simulink model "viswa9"  (Simulink 7.3)
settings: Solver=ode45  StartTime=0.0  StopTime=0.5  RelTol=1e-3
undefined symbols (not defined in the file): D11, Delta, Hydride, magnitude, Metal, Nickel
libraries: powerlib x34, powerlib_extras x3, electricdrivelib x2, powerlib_models x2, simulink x1
settings Model: Creator=KREST  LastModifiedBy=s padmaja

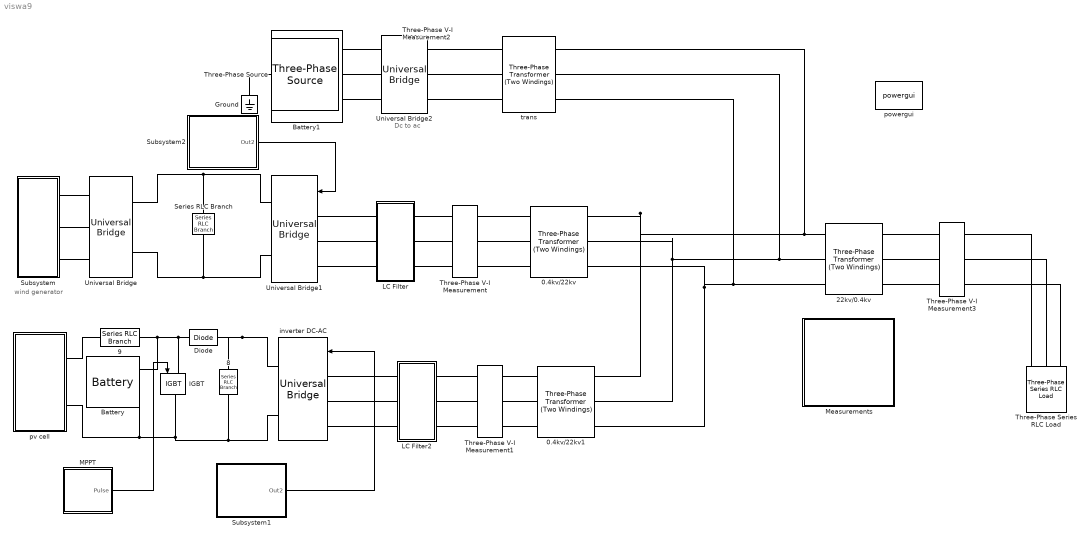
== system viswa9 ==
  note: Dc to ac
  note: wind generator
  0.4kv/22kv : powerlib/Elements/Three-Phase Transformer (Two Windings)  DialogController=POWERSYS.PowerSysDialog  SystemSampleTime=-1  Winding1Connection=Yg  UNITS=pu  NominalPower=[ 500e3 , 50 ]  Winding1=[ 0.4e3 , 0.002 , 0.08 ]  Winding2Connection=Delta (D11)  Winding2=[ 22e3 , 0.002 , 0.08 ]  SetSaturation=off  Rm=500  Lm=500  Saturation=[ 0,0 ; 0.0024,1.2 ; 1.0,1.52 ]  Hysteresis=off  DataFile='hysteresis'  SetInitialFlux=off  InitialFluxes=[ 0.8 , -0.8 , 0.7 ]  Measurements=None  MoreParameters=off  BreakLoop=off  DataType=off  TransfoNumber=1
  0.4kv/22kv1 : powerlib/Elements/Three-Phase Transformer (Two Windings)  DialogController=POWERSYS.PowerSysDialog  SystemSampleTime=-1  Winding1Connection=Yg  UNITS=pu  NominalPower=[ 500e3 , 50 ]  Winding1=[ 0.4e3 , 0.002 , 0.08 ]  Winding2Connection=Delta (D11)  Winding2=[ 22e3 , 0.002 , 0.08 ]  SetSaturation=off  Rm=500  Lm=500  Saturation=[ 0,0 ; 0.0024,1.2 ; 1.0,1.52 ]  Hysteresis=off  DataFile='hysteresis'  SetInitialFlux=off  InitialFluxes=[ 0.8 , -0.8 , 0.7 ]  Measurements=None  MoreParameters=off  BreakLoop=off  DataType=off  TransfoNumber=1
  22kv/0.4kv : powerlib/Elements/Three-Phase Transformer (Two Windings)  DialogController=POWERSYS.PowerSysDialog  SystemSampleTime=-1  Winding1Connection=Delta (D11)  UNITS=pu  NominalPower=[ 500e3 , 50 ]  Winding1=[ 0.4e3 , 0.002 , 0.08 ]  Winding2Connection=Yg  Winding2=[ 22e3 , 0.002 , 0.08 ]  SetSaturation=off  Rm=500  Lm=500  Saturation=[ 0,0 ; 0.0024,1.2 ; 1.0,1.52 ]  Hysteresis=off  DataFile='hysteresis'  SetInitialFlux=off  InitialFluxes=[ 0.8 , -0.8 , 0.7 ]  Measurements=None  MoreParameters=off  BreakLoop=off  DataType=off  TransfoNumber=1
  8 : powerlib/Elements/Series RLC Branch  DialogController=POWERSYS.PowerSysDialog  PhysicalDomain=powersysdomain  SubClassName=unknown  LeftPortType=p1  RightPortType=p1  LConnTagsString=__new0  RConnTagsString=__new0  BranchType=C  Resistance=1  Inductance=1e-3  SetiL0=off  InitialCurrent=0  Capacitance=1e-6  Setx0=off  InitialVoltage=0  Measurements=None
  9 : powerlib/Elements/Series RLC Branch  DialogController=POWERSYS.PowerSysDialog  PhysicalDomain=powersysdomain  SubClassName=unknown  LeftPortType=p1  RightPortType=p1  LConnTagsString=__new0  RConnTagsString=__new0  BranchType=L  Resistance=1  Inductance=1e-3  SetiL0=off  InitialCurrent=0  Capacitance=1e-6  Setx0=off  InitialVoltage=0  Measurements=None
  Battery : electricdrivelib/Extra Sources/Battery  SystemSampleTime=-1  BatType=Nickel-Metal-Hydride  ShowDetailedParameters=off  NomV=1.2  NomQ=1.5  SOC=100  PresetModel=off  MaxQ=1.575  FullV=0.016963  Dis_rate=0.0045  R=0.008  Normal_OP=0.021635  expZone="[0.01562      0.0045]"  Dis_Char=off  current=[1.5 3]  Units=Ampere-hour  Batt_Tr=30
  Battery1 : electricdrivelib/Extra Sources/Battery  SystemSampleTime=-1  BatType=Nickel-Metal-Hydride  ShowDetailedParameters=off  NomV=1.2  NomQ=1.5  SOC=100  PresetModel=off  MaxQ=1.575  FullV=0.016963  Dis_rate=0.0045  R=0.008  Normal_OP=0.021635  expZone="[0.01562      0.0045]"  Dis_Char=off  current=[1.5 3]  Units=Ampere-hour  Batt_Tr=30
  Diode : powerlib/Power Electronics/Diode  DialogController=POWERSYS.PowerSysDialog  SystemSampleTime=-1  Ron=0.001  Lon=0  Vf=0.8  IC=0  UseSnubber=off  Rs=500  Cs=250e-9  Measurements=off
  Ground : powerlib/Elements/Ground  DialogController=POWERSYS.PowerSysDialog  PhysicalDomain=powersysdomain  SubClassName=unknown  LeftPortType=p1  RightPortType=p1  LConnTagsString=a
  IGBT : powerlib/Power Electronics/IGBT  DialogController=POWERSYS.PowerSysDialog  SystemSampleTime=-1  Ron=0.001  Lon=0  Vf=1  Tf=1e-6  Tt=2e-6  IC=0  Rs=1e5  Cs=inf  Measurements=off
  LC Filter : Subsystem
  LC Filter2 : Subsystem
  MPPT : Subsystem
  Measurements : Subsystem
  Series RLC Branch : powerlib/Elements/Series RLC Branch  DialogController=POWERSYS.PowerSysDialog  PhysicalDomain=powersysdomain  SubClassName=unknown  LeftPortType=p1  RightPortType=p1  LConnTagsString=__new0  RConnTagsString=__new0  BranchType=C  Resistance=1  Inductance=1e-3  SetiL0=off  InitialCurrent=0  Capacitance=600e-6  Setx0=off  InitialVoltage=0  Measurements=None
  Subsystem : Subsystem
  Subsystem1 : Subsystem
  Subsystem2 : Subsystem
  Three-Phase Series RLC Load : powerlib/Elements/Three-Phase Series RLC Load  DialogController=POWERSYS.PowerSysDialog  PhysicalDomain=powersysdomain  SubClassName=unknown  LeftPortType=p1  RightPortType=p1  LConnTagsString=A|B|C  Configuration=Y (grounded)  NominalVoltage=380  NominalFrequency=50  ActivePower=500e3  InductivePower=0  CapacitivePower=0  Measurements=None
  Three-Phase V-I Measurement : powerlib/Measurements/Three-Phase V-I Measurement  DialogController=POWERSYS.PowerSysDialog  SystemSampleTime=-1  VoltageMeasurement=phase-to-ground  SetLabelV=on  LabelV=Vhabc  Vpu=off  CurrentMeasurement=yes  SetLabelI=on  LabelI=Ihabc  Ipu=off  Pbase=100e6  Vbase=500e3  OutputType=Complex  PhasorSimulation=off  PSBequivalent=0
  Three-Phase V-I Measurement1 : powerlib/Measurements/Three-Phase V-I Measurement  DialogController=POWERSYS.PowerSysDialog  SystemSampleTime=-1  VoltageMeasurement=phase-to-ground  SetLabelV=on  LabelV=Vpvabc  Vpu=off  CurrentMeasurement=yes  SetLabelI=on  LabelI=Ipvabc  Ipu=off  Pbase=100e6  Vbase=500e3  OutputType=Complex  PhasorSimulation=off  PSBequivalent=0
  Three-Phase V-I Measurement2 : powerlib/Measurements/Three-Phase V-I Measurement  DialogController=POWERSYS.PowerSysDialog  SystemSampleTime=-1  VoltageMeasurement=phase-to-ground  SetLabelV=on  LabelV=VEabc  Vpu=off  CurrentMeasurement=yes  SetLabelI=on  LabelI=IEabc  Ipu=off  Pbase=100e6  Vbase=500e3  OutputType=Complex  PhasorSimulation=off  PSBequivalent=0
  Three-Phase V-I Measurement3 : powerlib/Measurements/Three-Phase V-I Measurement  DialogController=POWERSYS.PowerSysDialog  SystemSampleTime=-1  VoltageMeasurement=phase-to-ground  SetLabelV=on  LabelV=Vlabc  Vpu=off  CurrentMeasurement=yes  SetLabelI=on  LabelI=Ilabc  Ipu=off  Pbase=100e6  Vbase=500e3  OutputType=Complex  PhasorSimulation=off  PSBequivalent=0
  Three-Phase Source : powerlib/Electrical Sources/Three-Phase Source  DialogController=POWERSYS.PowerSysDialog  SystemSampleTime=-1  Voltage=132e3  PhaseAngle=0  Frequency=50  InternalConnection=Yn  SpecifyImpedance=on  Resistance=0.8929  Inductance=16.58e-3  ShortCircuitLevel=100e6  BaseVoltage=22e3  XRratio=7
  Universal Bridge : powerlib/Power Electronics/Universal Bridge  DialogController=POWERSYS.PowerSysDialog  SystemSampleTime=-1  Arms=3  SnubberResistance=1e5  SnubberCapacitance=inf  Device=Diodes  Ron=1e-3  Lon=0  ForwardVoltages="[  0  0  ]"  ForwardVoltage=0  GTOparameters=[ 10e-6 , 20e-6 ]  IGBTparameters=[ 1e-6 , 2e-6 ]  Measurements=None  Measurements_2=None  converterType=Rectifier
  Universal Bridge1 : powerlib/Power Electronics/Universal Bridge  DialogController=POWERSYS.PowerSysDialog  SystemSampleTime=-1  Arms=3  SnubberResistance=1e5  SnubberCapacitance=inf  Device=IGBT / Diodes  Ron=1e-3  Lon=0  ForwardVoltages="[  0  0  ]"  ForwardVoltage=0  GTOparameters=[ 10e-6 , 20e-6 ]  IGBTparameters=[ 1e-6 , 2e-6 ]  Measurements=None  Measurements_2=None  converterType=Rectifier
  Universal Bridge2 : powerlib/Power Electronics/Universal Bridge  DialogController=POWERSYS.PowerSysDialog  SystemSampleTime=-1  Arms=3  SnubberResistance=1e5  SnubberCapacitance=inf  Device=Diodes  Ron=1e-3  Lon=0  ForwardVoltages="[  0  0  ]"  ForwardVoltage=0  GTOparameters=[ 10e-6 , 20e-6 ]  IGBTparameters=[ 1e-6 , 2e-6 ]  Measurements=None  Measurements_2=None  converterType=Rectifier
  inverter DC-AC : powerlib/Power Electronics/Universal Bridge  DialogController=POWERSYS.PowerSysDialog  SystemSampleTime=-1  Arms=3  SnubberResistance=1e5  SnubberCapacitance=inf  Device=IGBT / Diodes  Ron=1e-3  Lon=0  ForwardVoltages="[  0  0  ]"  ForwardVoltage=0  GTOparameters=[ 10e-6 , 20e-6 ]  IGBTparameters=[ 1e-6 , 2e-6 ]  Measurements=None  Measurements_2=None  converterType=Rectifier
  powergui : powerlib/powergui  Priority=1  SystemSampleTime=-1  SimulationMode=Discrete  SampleTime=1e-6  frequency=60  SPID=off  DisableSnubberDevices=off  DisableRonSwitches=off  DisableVfSwitches=off  SwTol=0  Interpol=off  frequencyindice=0  echomessages=off  HookPort=off  DisplayEquations=off  FunctionMessages=off  EnableUseOfTLC=off  x0status=blocks  RestoreLinks=warning  Frange=[0:2:500]  Ylog=off  Xlog=on  ShowGrid=off  save=off  variable=ZData  ZoomFFT=on  StartTime=0.0  cycles=1  DisplayStyle=1  fundamental=60  FreqAxis=off  MaxFrequency=1000  frequencyindicesteady=1  RmsSteady=1  display=off  Ts=0  methode=off
  pv cell : Subsystem
  trans : powerlib/Elements/Three-Phase Transformer (Two Windings)  DialogController=POWERSYS.PowerSysDialog  SystemSampleTime=-1  Winding1Connection=Yg  UNITS=pu  NominalPower=[ 500e3 , 50 ]  Winding1=[ 132e3 , 0.002 , 0.08 ]  Winding2Connection=Delta (D11)  Winding2=[ 22e3 , 0.002 , 0.08 ]  SetSaturation=off  Rm=500  Lm=500  Saturation=[ 0,0 ; 0.0024,1.2 ; 1.0,1.52 ]  Hysteresis=off  DataFile='hysteresis'  SetInitialFlux=off  InitialFluxes=[ 0.8 , -0.8 , 0.7 ]  Measurements=None  MoreParameters=off  BreakLoop=off  DataType=off  TransfoNumber=1
  wires:
  Subsystem2/1(Out2) -> Universal Bridge1/1
  Subsystem1/1(Out2) -> inverter DC-AC/1
  MPPT/1(Pulse) -> IGBT/1
  connections:
  Ground/LConn1 -- Three-Phase Source/LConn1
  Universal Bridge1/RConn1 -- Universal Bridge/RConn1 -- Series RLC Branch/LConn1
  Universal Bridge1/RConn2 -- Universal Bridge/RConn2 -- Series RLC Branch/RConn1
  Subsystem/RConn1 -- Universal Bridge/LConn1
  Subsystem/RConn2 -- Universal Bridge/LConn2
  Subsystem/RConn3 -- Universal Bridge/LConn3
  LC Filter/LConn1 -- Universal Bridge1/LConn1
  Universal Bridge1/LConn2 -- LC Filter/LConn2
  Universal Bridge1/LConn3 -- LC Filter/LConn3
  Three-Phase V-I Measurement/RConn2 -- 0.4kv/22kv/LConn2
  Three-Phase V-I Measurement/LConn2 -- LC Filter/RConn2
  LC Filter/RConn1 -- Three-Phase V-I Measurement/LConn1
  Three-Phase V-I Measurement/RConn1 -- 0.4kv/22kv/LConn1
  Three-Phase V-I Measurement/RConn3 -- 0.4kv/22kv/LConn3
  Three-Phase V-I Measurement/LConn3 -- LC Filter/RConn3
  inverter DC-AC/RConn2 -- 8/RConn1 -- IGBT/RConn1 -- pv cell/RConn2 -- Battery/LConn2
  pv cell/RConn1 -- 9/LConn1
  Diode/LConn1 -- IGBT/LConn1 -- 9/RConn1 -- Battery/LConn1
  LC Filter2/LConn2 -- inverter DC-AC/LConn2
  inverter DC-AC/LConn1 -- LC Filter2/LConn1
  LC Filter2/LConn3 -- inverter DC-AC/LConn3
  Three-Phase V-I Measurement1/LConn2 -- LC Filter2/RConn2
  LC Filter2/RConn1 -- Three-Phase V-I Measurement1/LConn1
  LC Filter2/RConn3 -- Three-Phase V-I Measurement1/LConn3
  Three-Phase V-I Measurement1/RConn2 -- 0.4kv/22kv1/LConn2
  Three-Phase V-I Measurement1/RConn1 -- 0.4kv/22kv1/LConn1
  Three-Phase V-I Measurement1/RConn3 -- 0.4kv/22kv1/LConn3
  trans/LConn2 -- Three-Phase V-I Measurement2/RConn2
  Three-Phase V-I Measurement2/RConn1 -- trans/LConn1
  trans/LConn3 -- Three-Phase V-I Measurement2/RConn3
  Three-Phase Source/RConn2 -- Three-Phase V-I Measurement2/LConn2
  Three-Phase Source/RConn1 -- Three-Phase V-I Measurement2/LConn1
  Three-Phase Source/RConn3 -- Three-Phase V-I Measurement2/LConn3
  Three-Phase V-I Measurement3/LConn2 -- 22kv/0.4kv/RConn2
  22kv/0.4kv/RConn1 -- Three-Phase V-I Measurement3/LConn1
  22kv/0.4kv/RConn3 -- Three-Phase V-I Measurement3/LConn3
  Three-Phase V-I Measurement3/RConn1 -- Three-Phase Series RLC Load/LConn1
  Three-Phase Series RLC Load/LConn2 -- Three-Phase V-I Measurement3/RConn2
  Three-Phase V-I Measurement3/RConn3 -- Three-Phase Series RLC Load/LConn3
  inverter DC-AC/RConn1 -- Diode/RConn1 -- 8/LConn1
  22kv/0.4kv/LConn1 -- 0.4kv/22kv/RConn1 -- 0.4kv/22kv1/RConn1 -- trans/RConn1
  0.4kv/22kv/RConn2 -- 0.4kv/22kv1/RConn2 -- 22kv/0.4kv/LConn2 -- trans/RConn2
  0.4kv/22kv/RConn3 -- 0.4kv/22kv1/RConn3 -- 22kv/0.4kv/LConn3 -- trans/RConn3

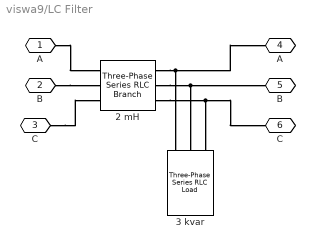
== system viswa9/LC Filter ==
  "2 mH " : powerlib/Elements/Three-Phase Series RLC Branch  DialogController=POWERSYS.PowerSysDialog  PhysicalDomain=powersysdomain  SubClassName=unknown  LeftPortType=p1  RightPortType=p1  LConnTagsString=A|B|C  RConnTagsString=A|B|C  BranchType=L  Resistance=1.0  Inductance=2e-3  Capacitance=1.0  Measurements=None
  3 kvar : powerlib/Elements/Three-Phase Series RLC Load  DialogController=POWERSYS.PowerSysDialog  PhysicalDomain=powersysdomain  SubClassName=unknown  LeftPortType=p1  RightPortType=p1  LConnTagsString=A|B|C  Configuration=Y (grounded)  NominalVoltage=380  NominalFrequency=50  ActivePower=0  InductivePower=0  CapacitivePower=3e3  Measurements=None
  A : PMIOPort  Port=1  Side=Left
  B : PMIOPort  Port=2  Side=Left
  C : PMIOPort  Port=3  Side=Left
  "A " : PMIOPort  Port=4  Side=Right
  "B " : PMIOPort  Port=5  Side=Right
  "C " : PMIOPort  Port=6  Side=Right
  connections:
  B/RConn1 -- "2 mH "/LConn2
  A/RConn1 -- "2 mH "/LConn1
  C/RConn1 -- "2 mH "/LConn3
  "2 mH "/RConn1 -- "A "/RConn1 -- 3 kvar/LConn1
  "2 mH "/RConn2 -- "B "/RConn1 -- 3 kvar/LConn2
  "2 mH "/RConn3 -- "C "/RConn1 -- 3 kvar/LConn3

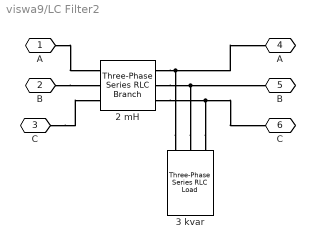
== system viswa9/LC Filter2 ==
  "2 mH " : powerlib/Elements/Three-Phase Series RLC Branch  DialogController=POWERSYS.PowerSysDialog  PhysicalDomain=powersysdomain  SubClassName=unknown  LeftPortType=p1  RightPortType=p1  LConnTagsString=A|B|C  RConnTagsString=A|B|C  BranchType=L  Resistance=1.0  Inductance=2e-3  Capacitance=1.0  Measurements=None
  3 kvar : powerlib/Elements/Three-Phase Series RLC Load  DialogController=POWERSYS.PowerSysDialog  PhysicalDomain=powersysdomain  SubClassName=unknown  LeftPortType=p1  RightPortType=p1  LConnTagsString=A|B|C  Configuration=Y (grounded)  NominalVoltage=380  NominalFrequency=50  ActivePower=0  InductivePower=0  CapacitivePower=3e3  Measurements=None
  A : PMIOPort  Port=1  Side=Left
  B : PMIOPort  Port=2  Side=Left
  C : PMIOPort  Port=3  Side=Left
  "A " : PMIOPort  Port=4  Side=Right
  "B " : PMIOPort  Port=5  Side=Right
  "C " : PMIOPort  Port=6  Side=Right
  connections:
  3 kvar/LConn3 -- "C "/RConn1 -- "2 mH "/RConn3
  3 kvar/LConn2 -- "B "/RConn1 -- "2 mH "/RConn2
  3 kvar/LConn1 -- "A "/RConn1 -- "2 mH "/RConn1
  C/RConn1 -- "2 mH "/LConn3
  A/RConn1 -- "2 mH "/LConn1
  B/RConn1 -- "2 mH "/LConn2

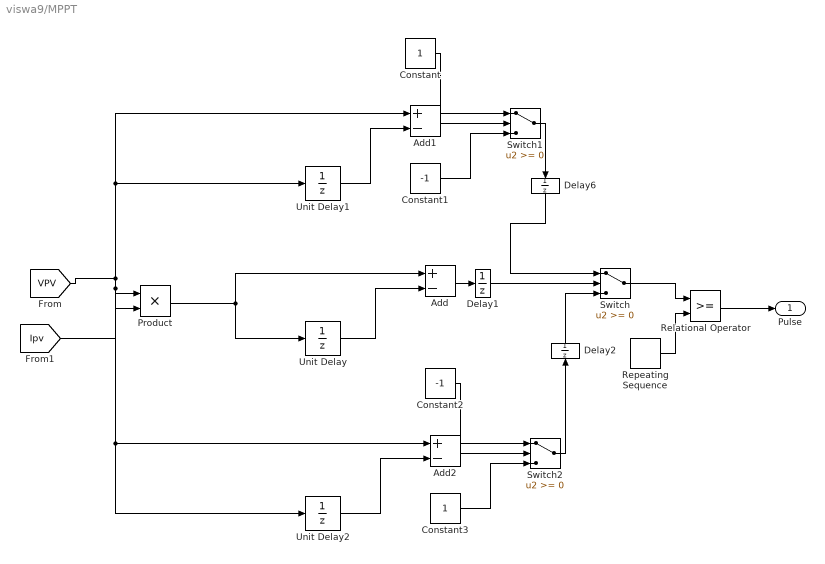
== system viswa9/MPPT ==
  Add : Sum  Inputs=+-  OutDataType=fixdt(1, 16)  OutScaling=2^-10
  Add1 : Sum  Inputs=+-  OutDataType=fixdt(1, 16)  OutScaling=2^-10
  Add2 : Sum  Inputs=+-  OutDataType=fixdt(1, 16)  OutScaling=2^-10
  Constant : Constant  OutDataType=fixdt(1, 16)  OutScaling=2^0
  Constant1 : Constant  Value=-1  OutDataType=fixdt(1, 16)  OutScaling=2^0
  Constant2 : Constant  Value=-1  OutDataType=fixdt(1, 16)  OutScaling=2^0
  Constant3 : Constant  OutDataType=fixdt(1, 16)  OutScaling=2^0
  Delay1 : UnitDelay  SampleTime=-1
  Delay2 : UnitDelay  SampleTime=-1
  Delay6 : UnitDelay  SampleTime=-1
  Product : Product  OutDataType=sfix(16)  OutScaling=2^0  RndMeth=Zero
  Relational Operator : RelationalOperator  LogicOutDataTypeMode=boolean  LogicDataType=fixdt(0, 8)  OutDataTypeStr=boolean
  Repeating Sequence : simulink/Sources/Repeating Sequence  SystemSampleTime=-1  rep_seq_t=[0 1/1500/4 3/1500/4 1/1500]  rep_seq_y=[0 1 -1 0]
  Switch : Switch  OutDataType=fixdt(1, 16)  OutScaling=2^0
  Switch1 : Switch  OutDataType=fixdt(1, 16)  OutScaling=2^0
  Switch2 : Switch  OutDataType=fixdt(1, 16)  OutScaling=2^0
  Unit Delay : UnitDelay  SampleTime=50e-6
  Unit Delay1 : UnitDelay  SampleTime=50e-6
  Unit Delay2 : UnitDelay  SampleTime=50e-6
  Pulse : Outport  OutDataType=sfix(16)  OutScaling=2^0
  wires:
  [VPV] -> Add1/1, Unit Delay1/1, Product/1, Add2/1, Unit Delay2/1
  [Ipv] -> Product/2
  Product/1 -> Unit Delay/1, Add/1
  Unit Delay/1 -> Add/2
  Add/1 -> Delay1/1
  Switch1/1 -> Delay6/1
  Unit Delay1/1 -> Add1/2
  Add1/1 -> Switch1/2
  Constant/1 -> Switch1/1
  Constant1/1 -> Switch1/3
  Add2/1 -> Switch2/2
  Constant2/1 -> Switch2/1
  Constant3/1 -> Switch2/3
  Unit Delay2/1 -> Add2/2
  Switch2/1 -> Delay2/1
  Switch/1 -> Relational Operator/1
  Repeating Sequence/1 -> Relational Operator/2
  Relational Operator/1 -> Pulse/1
  Delay6/1 -> Switch/1
  Delay1/1 -> Switch/2
  Delay2/1 -> Switch/3

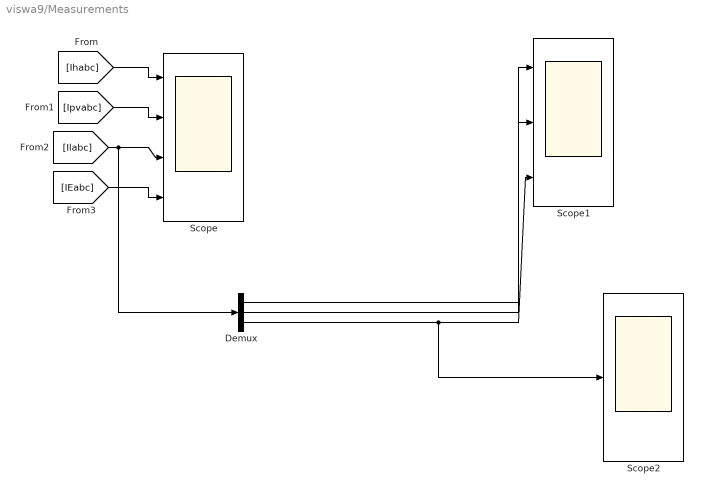
== system viswa9/Measurements ==
  Demux : Demux  Outputs=3
  Scope : Scope  NumInputPorts=4
      settings: YMin=4.75~5.65~-1.5~-15  YMax=7.75~6.25~2.5~20
  Scope1 : Scope  NumInputPorts=3
      settings: YMin=1.25~-2.1~0.05  YMax=1.8~-1.85~0.85
  Scope2 : Scope
      settings: YMin=-1.975  YMax=-1.7  SaveName=ScopeData2
  wires:
  [Ihabc] -> Scope/1
  [Ipvabc] -> Scope/2
  [Ilabc] -> Scope/3, Demux/1
  [IEabc] -> Scope/4
  Demux/1 -> Scope1/1
  Demux/2 -> Scope1/2
  Demux/3 -> Scope1/3, Scope2/1

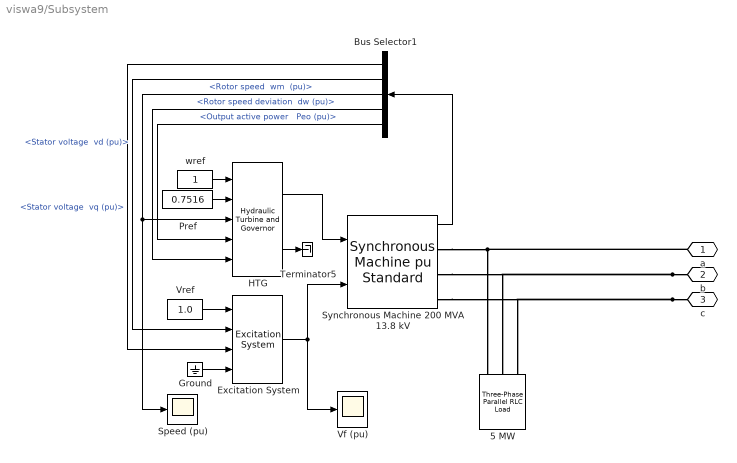
== system viswa9/Subsystem ==
  " Speed (pu)" : Scope
      settings: TickLabels=on  TimeRange=2  YMin=0.98  YMax=1.02  SaveName=Pm  DataFormat=Array
  5 MW : powerlib/Elements/Three-Phase Parallel RLC Load  DialogController=POWERSYS.PowerSysDialog  PhysicalDomain=powersysdomain  SubClassName=unknown  LeftPortType=p1  RightPortType=p1  LConnTagsString=A|B|C  Configuration=Y (grounded)  NominalVoltage=380  NominalFrequency=50  ActivePower=5e3  InductivePower=0  CapacitivePower=0  Measurements=None
  Bus Selector1 : BusSelector  OutputSignals="dq0 components.Stator voltage  vq (pu),dq0 components.Stator voltage  vd (pu),Mechanical.Rotor speed  wm  (pu),Mechanical.Rotor speed deviation  dw (pu),Output active power   Peo (pu)"
  Excitation System : powerlib/Machines/Excitation System  DialogController=POWERSYS.PowerSysDialog  SystemSampleTime=-1  tr=20e-3  reg=[ 300, 0.001 ]  exc=[ 1, 0 ]  tgr=[ 0, 0 ]  damp=[ 0.001, 0.1 ]  sat=[ 0, 0 ]  lim=[ -11.5, 11.5, 0 ]  v0=[1,1.0]
  Ground : Ground
  HTG : powerlib/Machines/Hydraulic Turbine and Governor  DialogController=POWERSYS.PowerSysDialog  SystemSampleTime=-1  sm="[ 10/3  0.07 ]"  gate="[  0.01  0.97518  -0.1  0.1 ]"  reg="[  0.05  1.163  0.105  0  0.01  ]"  hyd="[  0  2.67  ]"  dref=0  po=1
  Pref : Constant  Value=0.7516  OutDataType=sfix(16)  OutScaling=2^0
  Synchronous Machine 200 MVA 13.8 kV : powerlib/Machines/Synchronous Machine pu Standard  DialogController=POWERSYS.PowerSysDialog  SystemSampleTime=-1  PresetModel=No  MechanicalLoad=Mechanical power Pm  ShowDetailedParameters=on  RotorType=Salient-pole  NominalParameters="[ 1000e3  380   50 ]"  Reactances1=[ 31 32 33 34 35 36 37 ]  Reactances2=[ 1.305, 0.296, 0.252, 0.474, 0.243, 0.18 ]  dAxisTimeConstants=Short-circuit  qAxisTimeConstants=Open-circuit  TimeConstants1=[]  TimeConstants2=[]  TimeConstants3=[]  TimeConstants4=[]  TimeConstants5=[ 1.01, 0.053, 0.1 ]  TimeConstants6=[]  TimeConstants7=[]  TimeConstants8=[]  StatorResistance=2.8544e-3  Mechanical="[ 3.2 0  32]"  PolePairs=32  InitialConditions=[0 0 0 0 0 0 0 0 1]  SetSaturation=off  Saturation=[0.6404,0.7127,0.8441,0.9214,0.9956,1.082,1.19,1.316,1.457;0.7,0.7698,0.8872,0.9466,0.9969,1.046,1.1,1.151,1.201]  Units=per unit standard parameters  LoadFlowParameters=[1 150000000 0 0]  TsPowergui=0  TsBlock=-1  IterativeModel=Forward Euler
      settings: AttributesFormatString=\n\n
  Terminator5 : Terminator
  Vf (pu) : Scope
      settings: TickLabels=on  TimeRange=2  YMin=-10  YMax=15  SaveName=vf  DataFormat=Array
  Vref : Constant  Value=1.0  OutDataType=sfix(16)  OutScaling=2^0
  wref : Constant  OutDataType=sfix(16)  OutScaling=2^0
  a : PMIOPort  Port=1  Side=Right
  b : PMIOPort  Port=2  Side=Right
  c : PMIOPort  Port=3  Side=Right
  wires:
  Ground/1 -> Excitation System/4
  HTG/2 -> Terminator5/1
  Vref/1 -> Excitation System/1
  Pref/1 -> HTG/2
  wref/1 -> HTG/1
  Excitation System/1 -> Vf (pu)/1, Synchronous Machine 200 MVA 13.8 kV/2
  HTG/1 -> Synchronous Machine 200 MVA 13.8 kV/1
  Bus Selector1/1 -> Excitation System/3  "<Stator voltage  vq (pu)>"
  Bus Selector1/2 -> Excitation System/2  "<Stator voltage  vd (pu)>"
  Bus Selector1/3 -> HTG/3, " Speed (pu)"/1  "<Rotor speed  wm  (pu)>"
  Bus Selector1/4 -> HTG/5  "<Rotor speed deviation  dw (pu)>"
  Bus Selector1/5 -> HTG/4  "<Output active power   Peo (pu)>"
  Synchronous Machine 200 MVA 13.8 kV/1 -> Bus Selector1/1
  connections:
  b/RConn1 -- Synchronous Machine 200 MVA 13.8 kV/RConn2 -- 5 MW/LConn2
  c/RConn1 -- Synchronous Machine 200 MVA 13.8 kV/RConn3 -- 5 MW/LConn3
  a/RConn1 -- Synchronous Machine 200 MVA 13.8 kV/RConn1 -- 5 MW/LConn1

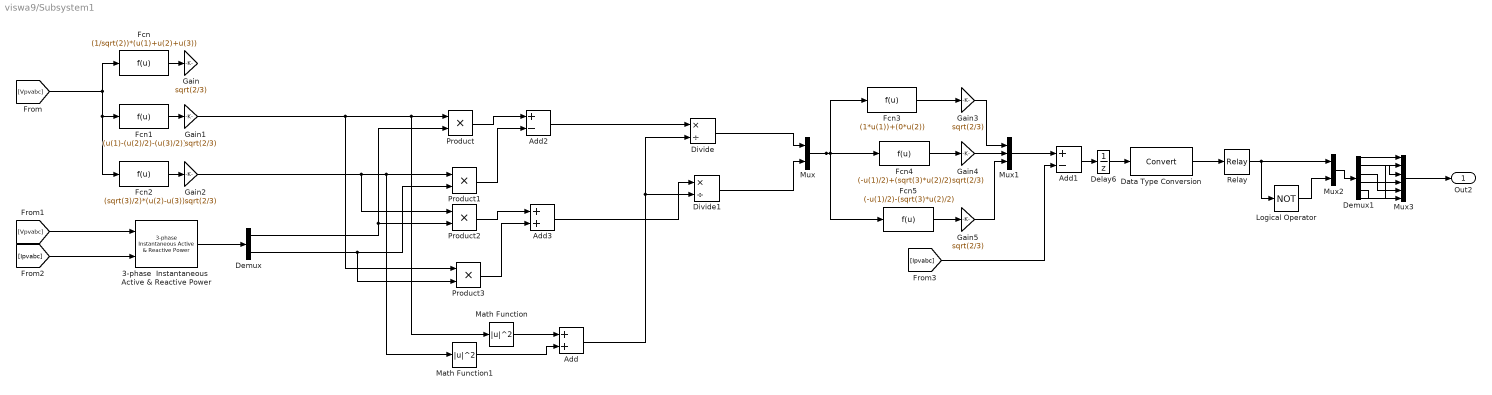
== system viswa9/Subsystem1 ==
  3-phase  Instantaneous  Active & Reactive Power : powerlib_extras/Measurements/3-phase  Instantaneous  Active & Reactive Power  DialogController=POWERSYS.PowerSysDialog  SystemSampleTime=-1
  Add : Sum  OutDataType=fixdt(1, 16)  OutScaling=2^-10
  Add1 : Sum  Inputs=+-  OutDataType=fixdt(1, 16)  OutScaling=2^-10
  Add2 : Sum  Inputs=+-  OutDataType=fixdt(1, 16)  OutScaling=2^-10
  Add3 : Sum  OutDataType=fixdt(1, 16)  OutScaling=2^-10
  Data Type Conversion : DataTypeConversion  OutDataType=fixdt(1, 16)  OutScaling=2^0
  Delay6 : UnitDelay  SampleTime=-1
  Demux : Demux  Outputs=2
  Demux1 : Demux  Outputs=6
  Divide : Product  Inputs=*/  OutDataType=fixdt(1, 16)  OutScaling=2^-10
  Divide1 : Product  Inputs=*/  OutDataType=fixdt(1, 16)  OutScaling=2^-10
  Fcn : Fcn  Expr=(1/sqrt(2))*(u(1)+u(2)+u(3))
  Fcn1 : Fcn  Expr=(u(1)-(u(2)/2)-(u(3)/2))
  Fcn2 : Fcn  Expr=(sqrt(3)/2)*(u(2)-u(3))
  Fcn3 : Fcn  Expr=(1*u(1))+(0*u(2))
  Fcn4 : Fcn  Expr=(-u(1)/2)+(sqrt(3)*u(2)/2)
  Fcn5 : Fcn  Expr=(-u(1)/2)-(sqrt(3)*u(2)/2)
  Gain{,1..5} (6 alike) : Gain  Gain=sqrt(2/3)  ParameterDataType=fixdt(1, 16)  ParameterScaling=2^0  OutDataType=fixdt(1, 16)  OutScaling=2^0
  Logical Operator : Logic  Operator=NOT  AllPortsSameDT=off  OutDataTypeMode=boolean  LogicDataType=fixdt(0, 8)  OutDataTypeStr=boolean
  Math Function : Math  Operator=magnitude^2  OutDataType=fixdt(1, 16)  OutScaling=2^0  SaturateOnIntegerOverflow=on
  Math Function1 : Math  Operator=magnitude^2  OutDataType=fixdt(1, 16)  OutScaling=2^0  SaturateOnIntegerOverflow=on
  Mux : Mux  Inputs=2
  Mux1 : Mux  Inputs=3
  Mux2 : Mux  Inputs=2
  Mux3 : Mux  Inputs=6
  Product{,1..3} (4 alike) : Product  OutDataType=fixdt(1, 16)  OutScaling=2^0  RndMeth=Zero
  Relay : Relay  OnSwitchValue=0.1  OffSwitchValue=-0.1  OutDataType=fixdt(1, 16)  OutScaling=2^0
  Out2 : Outport
  wires:
  Add3/1 -> Divide1/1
  Product3/1 -> Add3/2
  Product2/1 -> Add3/1
  Product1/1 -> Add2/2
  Product/1 -> Add2/1
  Add2/1 -> Divide/1
  [Vpvabc] -> Fcn/1, Fcn1/1, Fcn2/1
  Fcn/1 -> Gain/1
  Fcn1/1 -> Gain1/1
  Fcn2/1 -> Gain2/1
  Gain1/1 -> Product3/1, Product/1, Math Function/1
  Gain2/1 -> Product2/1, Product1/1, Math Function1/1
  [Vpvabc] -> 3-phase  Instantaneous  Active & Reactive Power/1
  [Ipvabc] -> 3-phase  Instantaneous  Active & Reactive Power/2
  3-phase  Instantaneous  Active & Reactive Power/1 -> Demux/1
  Demux/1 -> Product2/2, Product/2
  Demux/2 -> Product3/2, Product1/2
  Math Function/1 -> Add/1
  Math Function1/1 -> Add/2
  Add/1 -> Divide1/2, Divide/2
  Divide/1 -> Mux/1
  Divide1/1 -> Mux/2
  Mux/1 -> Fcn4/1, Fcn3/1, Fcn5/1
  Fcn3/1 -> Gain3/1
  Fcn4/1 -> Gain4/1
  Fcn5/1 -> Gain5/1
  Gain3/1 -> Mux1/1
  Gain4/1 -> Mux1/2
  Gain5/1 -> Mux1/3
  Mux1/1 -> Add1/1
  [Ipvabc] -> Add1/2
  Add1/1 -> Delay6/1
  Relay/1 -> Logical Operator/1, Mux2/1
  Logical Operator/1 -> Mux2/2
  Mux2/1 -> Demux1/1
  Mux3/1 -> Out2/1
  Demux1/1 -> Mux3/1
  Demux1/2 -> Mux3/3
  Demux1/3 -> Mux3/5
  Demux1/4 -> Mux3/4
  Demux1/5 -> Mux3/6
  Demux1/6 -> Mux3/2
  Data Type Conversion/1 -> Relay/1
  Delay6/1 -> Data Type Conversion/1

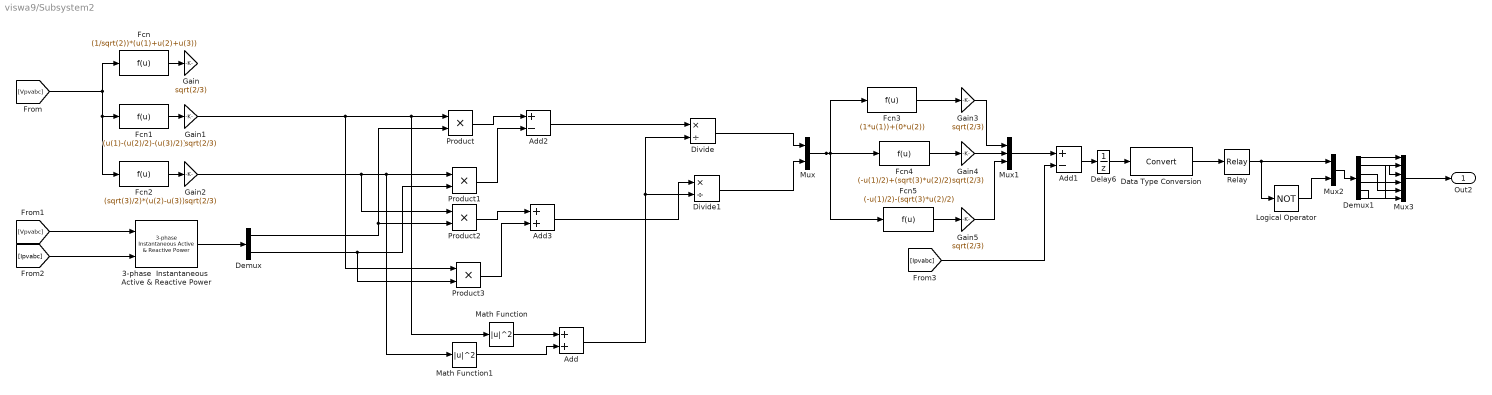
== system viswa9/Subsystem2 ==
  3-phase  Instantaneous  Active & Reactive Power : powerlib_extras/Measurements/3-phase  Instantaneous  Active & Reactive Power  DialogController=POWERSYS.PowerSysDialog  SystemSampleTime=-1
  Add : Sum  OutDataType=fixdt(1, 16)  OutScaling=2^-10
  Add1 : Sum  Inputs=+-  OutDataType=fixdt(1, 16)  OutScaling=2^-10
  Add2 : Sum  Inputs=+-  OutDataType=fixdt(1, 16)  OutScaling=2^-10
  Add3 : Sum  OutDataType=fixdt(1, 16)  OutScaling=2^-10
  Data Type Conversion : DataTypeConversion  OutDataType=fixdt(1, 16)  OutScaling=2^0
  Delay6 : UnitDelay  SampleTime=-1
  Demux : Demux  Outputs=2
  Demux1 : Demux  Outputs=6
  Divide : Product  Inputs=*/  OutDataType=fixdt(1, 16)  OutScaling=2^-10
  Divide1 : Product  Inputs=*/  OutDataType=fixdt(1, 16)  OutScaling=2^-10
  Fcn : Fcn  Expr=(1/sqrt(2))*(u(1)+u(2)+u(3))
  Fcn1 : Fcn  Expr=(u(1)-(u(2)/2)-(u(3)/2))
  Fcn2 : Fcn  Expr=(sqrt(3)/2)*(u(2)-u(3))
  Fcn3 : Fcn  Expr=(1*u(1))+(0*u(2))
  Fcn4 : Fcn  Expr=(-u(1)/2)+(sqrt(3)*u(2)/2)
  Fcn5 : Fcn  Expr=(-u(1)/2)-(sqrt(3)*u(2)/2)
  Gain{,1..5} (6 alike) : Gain  Gain=sqrt(2/3)  ParameterDataType=fixdt(1, 16)  ParameterScaling=2^0  OutDataType=fixdt(1, 16)  OutScaling=2^0
  Logical Operator : Logic  Operator=NOT  AllPortsSameDT=off  OutDataTypeMode=boolean  LogicDataType=fixdt(0, 8)  OutDataTypeStr=boolean
  Math Function : Math  Operator=magnitude^2  OutDataType=fixdt(1, 16)  OutScaling=2^0  SaturateOnIntegerOverflow=on
  Math Function1 : Math  Operator=magnitude^2  OutDataType=fixdt(1, 16)  OutScaling=2^0  SaturateOnIntegerOverflow=on
  Mux : Mux  Inputs=2
  Mux1 : Mux  Inputs=3
  Mux2 : Mux  Inputs=2
  Mux3 : Mux  Inputs=6
  Product{,1..3} (4 alike) : Product  OutDataType=fixdt(1, 16)  OutScaling=2^0  RndMeth=Zero
  Relay : Relay  OnSwitchValue=0.1  OffSwitchValue=-0.1  OutDataType=fixdt(1, 16)  OutScaling=2^0
  Out2 : Outport
  wires:
  Delay6/1 -> Data Type Conversion/1
  Data Type Conversion/1 -> Relay/1
  Demux1/6 -> Mux3/2
  Demux1/5 -> Mux3/6
  Demux1/4 -> Mux3/4
  Demux1/3 -> Mux3/5
  Demux1/2 -> Mux3/3
  Demux1/1 -> Mux3/1
  Mux3/1 -> Out2/1
  Mux2/1 -> Demux1/1
  Logical Operator/1 -> Mux2/2
  Relay/1 -> Mux2/1, Logical Operator/1
  Add1/1 -> Delay6/1
  [Ipvabc] -> Add1/2
  Mux1/1 -> Add1/1
  Gain5/1 -> Mux1/3
  Gain4/1 -> Mux1/2
  Gain3/1 -> Mux1/1
  Fcn5/1 -> Gain5/1
  Fcn4/1 -> Gain4/1
  Fcn3/1 -> Gain3/1
  Mux/1 -> Fcn5/1, Fcn3/1, Fcn4/1
  Divide1/1 -> Mux/2
  Divide/1 -> Mux/1
  Add/1 -> Divide/2, Divide1/2
  Math Function1/1 -> Add/2
  Math Function/1 -> Add/1
  Demux/2 -> Product1/2, Product3/2
  Demux/1 -> Product/2, Product2/2
  3-phase  Instantaneous  Active & Reactive Power/1 -> Demux/1
  [Ipvabc] -> 3-phase  Instantaneous  Active & Reactive Power/2
  [Vpvabc] -> 3-phase  Instantaneous  Active & Reactive Power/1
  Gain2/1 -> Math Function1/1, Product1/1, Product2/1
  Gain1/1 -> Math Function/1, Product/1, Product3/1
  Fcn2/1 -> Gain2/1
  Fcn1/1 -> Gain1/1
  Fcn/1 -> Gain/1
  [Vpvabc] -> Fcn2/1, Fcn1/1, Fcn/1
  Add2/1 -> Divide/1
  Product/1 -> Add2/1
  Product1/1 -> Add2/2
  Product2/1 -> Add3/1
  Product3/1 -> Add3/2
  Add3/1 -> Divide1/1

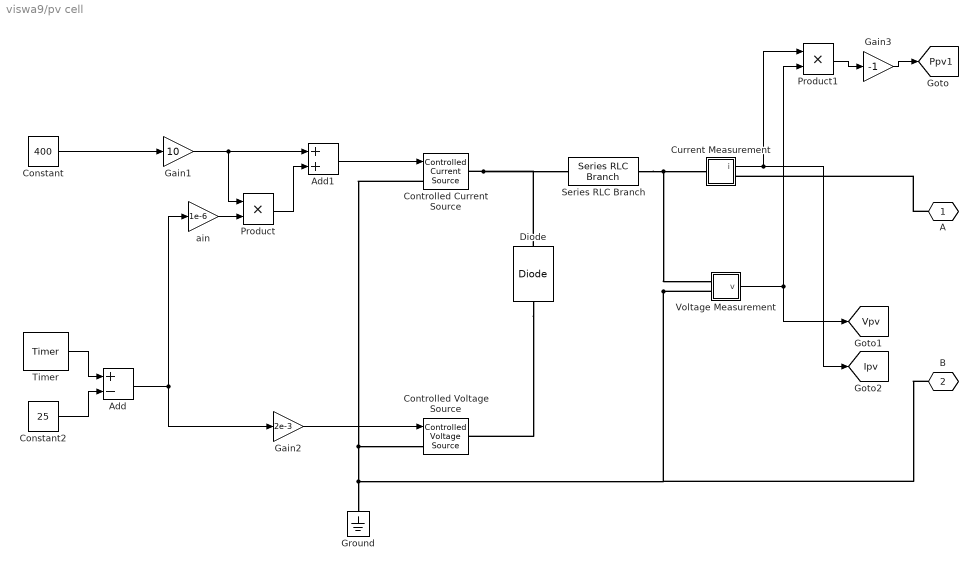
== system viswa9/pv cell ==
  Add : Sum  Inputs=+-  OutDataType=sfix(16)  OutScaling=2^-10  SampleTime=50e-6
  Add1 : Sum  OutDataType=sfix(16)  OutScaling=2^-10  SampleTime=50e-6
  Constant : Constant  Value=400  OutDataType=sfix(16)  OutScaling=2^0
  Constant2 : Constant  Value=25  OutDataType=sfix(16)  OutScaling=2^0
  Controlled Current Source : powerlib/Electrical Sources/Controlled Current Source  DialogController=POWERSYS.PowerSysDialog  SystemSampleTime=-1  Initialize=off  Source_Type=DC  Amplitude=0  Phase=0  Frequency=0  Measurements=None
  Controlled Voltage Source : powerlib/Electrical Sources/Controlled Voltage Source  DialogController=POWERSYS.PowerSysDialog  SystemSampleTime=-1  Initialize=off  Source_Type=DC  Amplitude=0  Phase=0  Frequency=0  Measurements=None
  Current Measurement : Subsystem  DialogController=POWERSYS.PowerSysDialog  mask(Current Measurement){PhasorSimulation=off, OutputType=Complex, PSBequivalent=0}
      mask prompts: PhasorSimulation "Phasor simulation"; OutputType "Output signal :"; PSBequivalent "Equivalent circuit"
      mask help: Ideal current measurement.
      mask init:
      | block = gcb;
      | powericon('psbloadfunction',block,'Measurement Block','Initialize');
      | powericon('MeasurementBlockInit',block);
      | power_initmask();
      settings: CopyFcn=powericon('psbloadfunction',gcb,'Measurement Block','UpdateGotoTag');
      settings: PreSaveFcn=|
      | if strcmp('inactive',get_param(gcb,'linkstatus'));
      | 
      | set_param(gcb,'Linkstatus','restore')
      | end
      mask Help: web(psbhelp);
      mask StyleString: checkbox,popup(Complex|Real-Imag|Magnitude-Angle|Magnitude),edit
  Diode : powerlib/Power Electronics/Diode  DialogController=POWERSYS.PowerSysDialog  SystemSampleTime=-1  Ron=0.001  Lon=0  Vf=0.8  IC=0  UseSnubber=off  Rs=500  Cs=250e-9  Measurements=off
  Gain1 : Gain  Gain=10  ParameterDataType=sfix(16)  ParameterScaling=2^0  OutDataType=sfix(16)  OutScaling=2^0  SampleTime=50e-6
  Gain2 : Gain  Gain=2e-3  ParameterDataType=sfix(16)  ParameterScaling=2^0  OutDataType=sfix(16)  OutScaling=2^0  SampleTime=50e-6
  Gain3 : Gain  Gain=-1  ParameterDataType=sfix(16)  ParameterScaling=2^0  OutDataType=sfix(16)  OutScaling=2^0  SampleTime=50e-6
  Ground : powerlib/Elements/Ground  DialogController=POWERSYS.PowerSysDialog  PhysicalDomain=powersysdomain  SubClassName=unknown  LeftPortType=p1  RightPortType=p1  LConnTagsString=a
  Product : Product  OutDataType=sfix(16)  OutScaling=2^0  SampleTime=50e-6  RndMeth=Zero
  Product1 : Product  OutDataType=sfix(16)  OutScaling=2^0  SampleTime=50e-6  RndMeth=Zero
  Series RLC Branch : powerlib/Elements/Series RLC Branch  DialogController=POWERSYS.PowerSysDialog  PhysicalDomain=powersysdomain  SubClassName=unknown  LeftPortType=p1  RightPortType=p1  LConnTagsString=__new0  RConnTagsString=__new0  BranchType=R  Resistance=8e-3  Inductance=1e-3  SetiL0=off  InitialCurrent=0  Capacitance=1e-6  Setx0=off  InitialVoltage=0  Measurements=None
  Timer : powerlib_extras/Control  Blocks/Timer  DialogController=POWERSYS.PowerSysDialog  SystemSampleTime=-1  t="[ 0  3  5  ]"  e="[45  55 60 ]"
  Voltage Measurement : Subsystem  DialogController=POWERSYS.PowerSysDialog  mask(Voltage Measurement){PhasorSimulation=off, OutputType=Complex, PSBequivalent=0}
      mask prompts: PhasorSimulation "Phasor simulation"; OutputType "Output signal :"; PSBequivalent "Equivalent circuit"
      mask help: Ideal voltage measurement.
      mask init:
      | block = gcb;
      | powericon('psbloadfunction',block,'Measurement Block','Initialize');
      | powericon('MeasurementBlockInit',block);
      | power_initmask();
      settings: CopyFcn=powericon('psbloadfunction',gcb,'Measurement Block','UpdateGotoTag');
      settings: PreSaveFcn=|
      | if strcmp('inactive',get_param(gcb,'linkstatus'));
      | 
      | set_param(gcb,'Linkstatus','restore')
      | end
      mask Help: web(psbhelp);
      mask StyleString: checkbox,popup(Complex|Real-Imag|Magnitude-Angle|Magnitude),edit
  ain : Gain  Gain=1e-6  ParameterDataType=sfix(16)  ParameterScaling=2^0  OutDataType=sfix(16)  OutScaling=2^0  SampleTime=50e-6
  A : PMIOPort  Tag=PMCPort  Port=1  Side=Right
  B : PMIOPort  Tag=PMCPort  Port=2  Side=Right
  tag scope: Ipv=global, Ppv1=global, Vpv=global
  wires:
  Timer/1 -> Add/1
  Constant2/1 -> Add/2
  Add/1 -> ain/1, Gain2/1
  Constant/1 -> Gain1/1
  Gain1/1 -> Add1/1, Product/1
  Product/1 -> Add1/2
  ain/1 -> Product/2
  Add1/1 -> Controlled Current Source/1
  Gain2/1 -> Controlled Voltage Source/1
  Voltage Measurement/1(v) -> Product1/2, [Vpv]
  Current Measurement/1(i) -> Product1/1, [Ipv]
  Product1/1 -> Gain3/1
  Gain3/1 -> [Ppv1]
  connections:
  Controlled Current Source/RConn1 -- Series RLC Branch/LConn1 -- Diode/LConn1
  Controlled Current Source/LConn1 -- Controlled Voltage Source/LConn1 -- Voltage Measurement/LConn2 -- B/RConn1 -- Ground/LConn1
  Series RLC Branch/RConn1 -- Voltage Measurement/LConn1 -- Current Measurement/LConn1
  Diode/RConn1 -- Controlled Voltage Source/RConn1
  A/RConn1 -- Current Measurement/RConn1

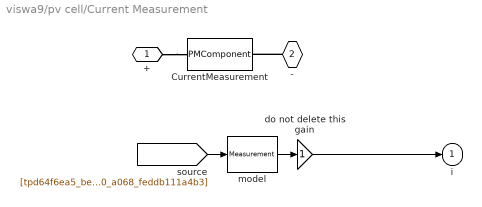
== system viswa9/pv cell/Current Measurement ==
  CurrentMeasurement : PMComponent  PhysicalDomain=powersysdomain  LeftPortType=p1  RightPortType=p1  LConnTagsString=a  RConnTagsString=__new0
      mask Type: InnerPowersysBlock
  do not delete this gain : Gain  ParameterDataType=sfix(16)  ParameterScaling=2^0  OutDataType=sfix(16)  OutScaling=2^0
  model : powerlib_models/Continuous/Measurement  SystemSampleTime=-1
  + : PMIOPort  Port=1  Side=Left
  - : PMIOPort  Port=2  Side=Right
  i : Outport  OutDataType=sfix(16)  OutScaling=2^0  InitialOutput=0
  wires:
  do not delete this gain/1 -> i/1
  model/1 -> do not delete this gain/1
  [tpd64f6ea5_bed7_4e90_a068_feddb111a4b3] -> model/1
  connections:
  +/RConn1 -- CurrentMeasurement/LConn1
  -/RConn1 -- CurrentMeasurement/RConn1

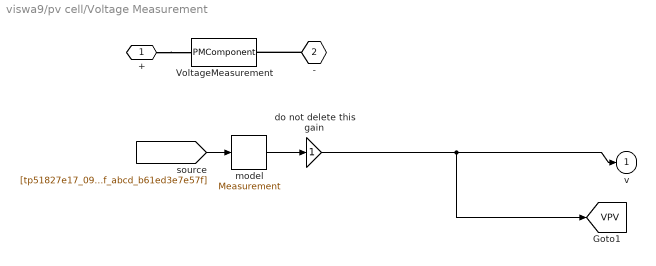
== system viswa9/pv cell/Voltage Measurement ==
  VoltageMeasurement : PMComponent  PhysicalDomain=powersysdomain  LeftPortType=p1  RightPortType=p1  LConnTagsString=+  RConnTagsString=-
      mask Type: InnerPowersysBlock
  do not delete this gain : Gain  ParameterDataType=sfix(16)  ParameterScaling=2^0  OutDataType=sfix(16)  OutScaling=2^0
  model : powerlib_models/Continuous/Measurement  SystemSampleTime=-1
  + : PMIOPort  Port=1  Side=Left
  - : PMIOPort  Port=2  Side=Left
  v : Outport  OutDataType=sfix(16)  OutScaling=2^0  InitialOutput=0
  tag scope: VPV=global
  wires:
  do not delete this gain/1 -> [VPV], v/1
  model/1 -> do not delete this gain/1
  [tp51827e17_0939_451f_abcd_b61ed3e7e57f] -> model/1
  connections:
  -/RConn1 -- VoltageMeasurement/RConn1
  +/RConn1 -- VoltageMeasurement/LConn1
